simulink subsystem "PvtSubSys_HMI"  (R2020b)
settings: Solver=VariableStepAuto  StartTime=0.0  StopTime=10.0  RelTol=1e-3
undefined symbols (not defined in the file): P_HMI_LDW_LKAWarnTime, P_HMI_ObjectTypeFilter, P_HMI_WarnFormLDWReq
libraries: simulink x212, TrueDurationTime x6
(part 7 of 8)

== matlab function PvtSubSys_HMI/HMI2.12/HWA//ACC//TJA_Signal1/MATLAB Function7 ==
  data: AngRaw input single; Angle output single
function Angle = AngCalc(AngRaw)
if AngRaw>1.57
    Angle = AngRaw - single(3.14);
elseif AngRaw<-1.57
    Angle = AngRaw + single(3.14);
else
    Angle = AngRaw;
end

== matlab function PvtSubSys_HMI/HMI2.12/HWA//ACC//TJA_Signal1/MATLAB Function8 ==
  data: Lane_ChangeReq input; LaneChange output
function LaneChange = fcn(Lane_ChangeReq)
LaneChange=uint8(0);
if Lane_ChangeReq==1
    LaneChange=uint8(1);
elseif Lane_ChangeReq==2
    LaneChange=uint8(2);
end

== matlab function PvtSubSys_HMI/HMI2.12/IFC_Signal1/MATLAB Function ==
  data: ELKState input; ELKmainState output
function ELKmainState  = fcn(ELKState)
ELKmainState=ELKState;
if ELKState == 3 || ELKState == 4
    ELKmainState = uint8(3);
elseif ELKState == 5 ||  ELKState == 6
    ELKmainState =uint8(4);
elseif ELKState == 7 ||  ELKState == 8
    ELKmainState = uint8(5);
elseif ELKState == 9
    ELKmainState = uint8(6);
end

== matlab function PvtSubSys_HMI/HMI2.12/IFC_Signal1/MATLAB Function1 ==
  data: fType input; Type output
function Type = fcn(fType)

Type=fType;
if fType==14||fType==20
    Type=uint8(2);
end

== matlab function PvtSubSys_HMI/HMI2.12/IFC_Signal1/MATLAB Function10 ==
  data: Lvalid input; y output; Rvalid input
function y = fcn(Lvalid,Rvalid)
if Lvalid>1 && Rvalid>1
  y=3;%double
elseif Lvalid>1 && Rvalid<2
    y=1 ; % left
elseif Lvalid<2 && Rvalid>1
    y=2; %right
else 
    y=0;
end

== matlab function PvtSubSys_HMI/HMI2.12/IFC_Signal1/MATLAB Function11 ==
  data: ELKSts input; LDW_LKAWarn output; LKAState input; Time input; count output; countk1 input
function [LDW_LKAWarn,count] = fcn(ELKSts,LKAState,Time,countk1)
count=0;
LDW_LKAWarn=uint8(0);
if ELKSts==uint8(3)||ELKSts==uint8(5)||ELKSts==uint8(7) || LKAState==uint8(4)
    count=countk1+1;
    if countk1>50*(Time-1)
        
        LDW_LKAWarn=uint8(1);
    end
elseif ELKSts==uint8(4)||ELKSts==uint8(6)||ELKSts==uint8(8) || LKAState==uint8(5)
    count=countk1+1;
    if countk1>50*(Time-1)
        LDW_LKAWarn=uint8(2);
    end
end

== matlab function PvtSubSys_HMI/HMI2.12/IFC_Signal1/Subsystem1/MATLAB Function3 ==
  data: Left_A0 input; Left_A1 input; Left_A2 input; Left_A3 input; L_A0 output; L_A1 output; L_A2 output; L_A3 output; Left_Type input; Left_Valid input; Right_A0 input; Right_A1 input; Right_A2 input; Right_A3 input; Right_Type input; Right_Valid input; LaneAvailability input; L_Type output uint8; L_Valid output uint8; R_A0 output; R_A1 output; R_A2 output; R_A3 output; R_Type output uint8; R_Valid output uint8
function [L_A0,L_A1,L_A2,L_A3,L_Type,L_Valid,R_A0,R_A1,R_A2,R_A3,R_Type,R_Valid] = LineCalc(Left_A0,Left_A1,Left_A2,Left_A3......
,Left_Type,Left_Valid,Right_A0,Right_A1,Right_A2,Right_A3,Right_Type,Right_Valid,LaneAvailability)
L_A0=single(0);
L_A1=single(0);
L_A2=single(0);
L_A3=single(0);
L_Type=uint8(0);
L_Valid=uint8(1);
R_A0=single(0);
R_A1=single(0);
R_A2=single(0);
R_A3=single(0);
R_Type=uint8(0);
R_Valid=uint8(1);

if LaneAvailability==1
    L_A0=Left_A0;
    L_A1=Left_A1;
    L_A2=Left_A2;
    L_A3=Left_A3;
    L_Type=Left_Type;
    L_Valid=Left_Valid;
elseif LaneAvailability==2
    R_A0=Right_A0;
    R_A1=Right_A1;
    R_A2=Right_A2;
    R_A3=Right_A3;
    R_Type=Right_Type;
    R_Valid=Right_Valid;
elseif LaneAvailability==3
    if abs(Left_A0-Right_A0)<5.5 && abs(Left_A0-Right_A0)>2.5
        L_A0=Left_A0;
        L_A1=Left_A1;
        L_A2=Left_A2;
        L_A3=Left_A3;
        L_Type=Left_Type;
        L_Valid=Left_Valid;
        R_A0=Right_A0;
        R_A1=Right_A1;
        R_A2=Right_A2;
        R_A3=Right_A3;
        R_Type=Right_Type;
        R_Valid=Right_Valid;
    elseif abs(Left_A0-Right_A0)>=5.5
        L_A0=5.5*Left_A0/abs(Left_A0-Right_A0);
        L_A1=Left_A1;
        L_A2=Left_A2;
        L_A3=Left_A3;
        L_Type=Left_Type;
        L_Valid=Left_Valid;
        R_A0=5.5*Right_A0/abs(Left_A0-Right_A0);
        R_A1=Right_A1;
        R_A2=Right_A2;
        R_A3=Right_A3;
        R_Type=Right_Type;
        R_Valid=Right_Valid;
    elseif abs(Left_A0-Right_A0)<=2.5&&abs(Left_A0-Right_A0)>0
        L_A0=2.5*Left_A0/abs(Left_A0-Right_A0);
        L_A1=Left_A1;
        L_A2=Left_A2;
        L_A3=Left_A3;
        L_Type=Left_Type;
        L_Valid=Left_Valid;
        R_A0=2.5*Right_A0/abs(Left_A0-Right_A0);
        R_A1=Right_A1;
        R_A2=Right_A2;
        R_A3=Right_A3;
        R_Type=Right_Type;
        R_Valid=Right_Valid;
    end
end

== matlab function PvtSubSys_HMI/HMI2.12/IFC_Signal1/MATLAB Function4 ==
  data: fType input; Type output
function Type = fcn(fType)

Type=fType;
if fType==14||fType==20
    Type=uint8(2);
end

== matlab function PvtSubSys_HMI/HMI2.12/IFC_Signal1/MATLAB Function5 ==
  data: fType input; Type output
function Type = fcn(fType)

Type=fType;
if fType==14||fType==20
    Type=uint8(2);
end

== matlab function PvtSubSys_HMI/HMI2.12/IFC_Signal1/Subsystem53/MATLAB Function1 ==
  data: standstill input boolean; out output single; in input single; update input boolean; inrecorder input single; recorder output single
function [out,recorder] = fcn(standstill,in,update,inrecorder)
recorder=inrecorder;
out=single(0);
if update%当车辆由运动到静止时记录recorder，并在车辆运动时将recorder清零
    recorder=in;
end
if standstill==0%车辆运动时采用实际值，车辆静止时采用recorder值
    out=in;
elseif standstill==1
    if update
        out=in;
    else
        out=inrecorder;
    end
end

== matlab function PvtSubSys_HMI/HMI2.12/IFC_Signal1/MATLAB Function7 ==
  data: ESSSts input; Intervention output; State output; Error output
function [Intervention,State,Error]  = fcn(ESSSts)

Intervention=uint8(0);
State=uint8(0);
Error=false;
if ESSSts>0
    State=uint8(1);
end
if ESSSts==4
    Intervention=uint8(1);
elseif ESSSts==5
    Intervention=uint8(2);
elseif ESSSts==6
    Error=true;
end

== matlab function PvtSubSys_HMI/HMI2.12/IFC_Signal1/MATLAB Function8 ==
  data: LDWActive input; LSSIntervention input; warnform input; WarnFormReq input; y output
function y = fcn(LDWActive, LSSIntervention,warnform, WarnFormReq)
y=uint8(0);
if (LSSIntervention==1 || LSSIntervention==2 || LSSIntervention==6 || LSSIntervention==7) && warnform==0
    if WarnFormReq==1 || WarnFormReq==2
        y=uint8(1);
    end
elseif (LSSIntervention==1 || LSSIntervention==2 || LSSIntervention==6 || LSSIntervention==7) && warnform==1
    if (WarnFormReq==1 || WarnFormReq==2) && LDWActive==true
        y=uint8(1);
    end   
end

== matlab function PvtSubSys_HMI/HMI2.12/IFC_Signal1/MATLAB Function9 ==
  data: ESSSts input; Intervention output; State output; Error output
function [Intervention,State,Error]  = fcn(ESSSts)

Intervention=uint8(0);
State=uint8(0);
Error=false;
if ESSSts>0
    State=uint8(1);
end
if ESSSts==4
    Intervention=uint8(1);
elseif ESSSts==5
    Intervention=uint8(2);
elseif ESSSts==6
    Error=true;
end

== matlab function PvtSubSys_HMI/HMI2.12/HWA//ACC//TJA_Signal1/MATLAB Function9 ==
  data: IntelligentCurveActive input boolean; y output uint8; ISL_InterSysInfoDisp input uint8; yk1 input uint8; countk1 input single; count output single
function [y,count] = fcn(IntelligentCurveActive, ISL_InterSysInfoDisp,yk1,countk1)

if yk1==uint8(3)
    count=single(6000);
else
    count=max(single(0),countk1-single(1));
end
if IntelligentCurveActive==true && count==single(0)
    y=uint8(3);
elseif ISL_InterSysInfoDisp==1 || ISL_InterSysInfoDisp==2 
    y=ISL_InterSysInfoDisp;
else
    y=uint8(0);
end

== matlab function PvtSubSys_HMI/HMI2.12/IFC_Signal1/Subsystem1/MATLAB Function2 ==
  data: LeftValid input; LaneAvailability output; RightValid input; LeftA0 input; RightA0 input
function LaneAvailability = fcn(LeftValid,RightValid,LeftA0,RightA0)
LaneAvailability=0;
if LeftValid==true && RightValid== true %% two lane
    LaneAvailability=3;
elseif LeftValid==true && RightValid==false %% left lane
    LaneAvailability=1;
elseif LeftValid==false && RightValid==true %% right lane
    LaneAvailability=2;
end

== matlab function PvtSubSys_HMI/HMI2.12/IFC_Signal1/Subsystem2/MATLAB Function ==
  data: Left_A0 input; L_A0 output; Left_Type input; Right_A0 input; Right_Type input; LaneAvailability input; L_Type output; R_A0 output; R_Type output
function [L_A0,L_Type,R_A0,R_Type] = fcn(Left_A0,Left_Type,Right_A0,Right_Type,LaneAvailability)
    L_A0=single(0);
    R_A0=single(0);
    L_Type=uint8(0);
    R_Type=uint8(0);
    
if LaneAvailability==1
    L_A0=Left_A0; 
    L_Type=Left_Type;
elseif LaneAvailability==2
    R_A0=Right_A0;
    R_Type=Right_Type;
elseif LaneAvailability==3
    L_A0=Left_A0;
    L_Type=Left_Type;
    R_A0=Right_A0;
    R_Type=Right_Type;
end

== matlab function PvtSubSys_HMI/HMI2.12/IFC_Signal1/Subsystem2/MATLAB Function2 ==
  data: LeftValid input; LeftA0 input; LaneAvailability output; RightValid input; RightA0 input
function LaneAvailability = fcn(LeftValid,LeftA0,RightValid,RightA0)

 LaneAvailability=0;
if LeftValid==true && RightValid== true %% two lane
    if LeftA0-RightA0>=5.5
        LaneAvailability=0;
        if LeftA0 < 2.75
            LaneAvailability=1;
        elseif RightA0> -2.75
            LaneAvailability=2;
        end
    elseif LeftA0-RightA0<5.5 && LeftA0-RightA0>2.5
         LaneAvailability=3;
    end
elseif LeftValid==true && RightValid==false %% left lane
    if LeftA0<2.75
        LaneAvailability=1;
    end
elseif LeftValid==false && RightValid==true %% right lane
    if RightA0>-2.75
         LaneAvailability=2;
    end
end

== matlab function PvtSubSys_HMI/HMI2.12/IFC_Signal1/MATLAB Function2 ==
  data: LSSSwtReq input; LDWState input; LKAState input; LCKState input; ELKSts input; LKAWarning input; LCKIESts input; TJAState input; LSS_WarnFormSwtReq input; LKASwtReq input; LCKSwtReq input; Lcountk1 input; LSSFuncSts output; LSSErrSts output; LSSResp output; LSSIntervention output; ELKResp output; LCKResp output; LKAResp output; LDWResp output; IntelligentEvaResp output; IntelligentEvaActSts output; Lcount output; Rcountk1 input; Rcount output
function [LSSFuncSts,LSSErrSts,LSSResp,LSSIntervention,ELKResp,LCKResp,LKAResp,LDWResp,......
    IntelligentEvaResp,IntelligentEvaActSts,Lcount,Rcount] = fcn( LSSSwtReq,LDWState,LKAState,LCKState,ELKSts,LKAWarning,LCKIESts,TJAState,LSS_WarnFormSwtReq,LKASwtReq,LCKSwtReq,Lcountk1,Rcountk1)
LSSIntervention=uint8(0);
LSSErrSts=uint8(0);
LSSResp=false;
LSSFuncSts=uint8(0);
ELKResp=false;
LCKResp=false;
LKAResp=false;
LDWResp=false;
IntelligentEvaResp=false;
IntelligentEvaActSts=uint8(0);
Lcount=50;
Rcount=50;


%% LSSSwtReq
if LSSSwtReq>0
     LSSResp=true;
end


%% LCKState
    if LCKState>0 && LCKSwtReq>0
        LCKResp=true;
        LSSFuncSts=uint8(3);
        if LCKState==3 && (ELKSts==0||ELKSts==1||ELKSts==2||ELKSts==9 || LKAState~=4 || LKAState~=5)
            LSSIntervention=uint8(5);
            if LKAWarning==1
                if LSS_WarnFormSwtReq==0 || LSS_WarnFormSwtReq==2
                LSSIntervention=uint8(1);
                elseif LSS_WarnFormSwtReq==1
                LSSIntervention=uint8(6);
                end
            elseif LKAWarning==2
               if LSS_WarnFormSwtReq==0 ||  LSS_WarnFormSwtReq==2
                  LSSIntervention=uint8(2);
               elseif LSS_WarnFormSwtReq==1
                LSSIntervention=uint8(7);
               end
            end
                
        elseif LCKState==7
            LSSErrSts=uint8(3);
        end
        
 %% LKAState
    elseif LKAState>0 &&  LKASwtReq>0
        LKAResp=true;
        LSSFuncSts=uint8(2);
        if LKAState==4 && (ELKSts==0||ELKSts==1||ELKSts==2||ELKSts==9)|| (Lcountk1>0&&Lcountk1<50)
            Lcount=max(0,Lcountk1-1);
            LSSIntervention=uint8(3);
            if LKAWarning==1 
                if LSS_WarnFormSwtReq==0 || LSS_WarnFormSwtReq==2
                LSSIntervention=uint8(1);
                elseif LSS_WarnFormSwtReq==1
                LSSIntervention=uint8(6);
                end
            end
        elseif LKAState==5 && (ELKSts==0||ELKSts==1||ELKSts==2||ELKSts==9)|| (Rcountk1>0&&Rcountk1<50)
            Rcount=max(0,Lcountk1-1);
            LSSIntervention=uint8(4);
            if LKAWarning==1
               if LSS_WarnFormSwtReq==0 ||  LSS_WarnFormSwtReq==2
                  LSSIntervention=uint8(2);
               elseif LSS_WarnFormSwtReq==1
                LSSIntervention=uint8(7);
               end
            end
        elseif LKAState==6
            LSSErrSts=uint8(2);
        end
%%  LDWState
    elseif LDWState>0
        LSSFuncSts=uint8(1);
        LDWResp=true;
        if LDWState==4 && (ELKSts==0||ELKSts==1||ELKSts==2||ELKSts==9|| LKAState~=4 || LKAState~=5)
            if LSS_WarnFormSwtReq==0 || LSS_WarnFormSwtReq==2
            LSSIntervention=uint8(1);
            elseif LSS_WarnFormSwtReq==1
                LSSIntervention=uint8(6);
            end
        elseif LDWState==5 && (ELKSts==0||ELKSts==1||ELKSts==2||ELKSts==9|| LKAState~=4 || LKAState~=5)
            if LSS_WarnFormSwtReq==0 ||  LSS_WarnFormSwtReq==2
            LSSIntervention=uint8(2);
            elseif LSS_WarnFormSwtReq==1
                LSSIntervention=uint8(7);
            end
        elseif LDWState==6 
            LSSErrSts=uint8(1);
        end   
    end
   

%% LCKIESwitch
if LCKIESts>0
    IntelligentEvaResp=true;
    if LCKIESts==4
        IntelligentEvaActSts=uint8(2);
    elseif LCKIESts==5
        IntelligentEvaActSts=uint8(1);
    end
end
%% ELKState
if ELKSts>0
   ELKResp=true;
   LSSFuncSts=uint8(2);
   if LCKState>0 && LCKSwtReq>0
       LSSFuncSts=uint8(3);
   end
    if ELKSts==5 || ELKSts==7 || ELKSts==3
            LSSIntervention=uint8(3);
            if LKAWarning==1
                if LSS_WarnFormSwtReq==0 || LSS_WarnFormSwtReq==2
                LSSIntervention=uint8(1);
                elseif LSS_WarnFormSwtReq==1
                LSSIntervention=uint8(6);
                end
            end
    elseif ELKSts==6 || ELKSts==8 || ELKSts==4
            LSSIntervention=uint8(4);
            if LKAWarning==1
               if LSS_WarnFormSwtReq==0 ||  LSS_WarnFormSwtReq==2
                  LSSIntervention=uint8(2);
               elseif LSS_WarnFormSwtReq==1
                LSSIntervention=uint8(7);
               end
            end
    elseif LKAState==4 || (Lcountk1>0&&Lcountk1<50)
         Lcount=max(0,Lcountk1-1);
            LSSIntervention=uint8(3);
            if LKAWarning==1 
                if LSS_WarnFormSwtReq==0 || LSS_WarnFormSwtReq==2
                LSSIntervention=uint8(1);
                elseif LSS_WarnFormSwtReq==1
                LSSIntervention=uint8(6);
                end
            end
    elseif LKAState==5 || (Rcountk1>0&&Rcountk1<50)
        Rcount=max(0,Lcountk1-1);
            LSSIntervention=uint8(4);
            if LKAWarning==1
               if LSS_WarnFormSwtReq==0 ||  LSS_WarnFormSwtReq==2
                  LSSIntervention=uint8(2);
               elseif LSS_WarnFormSwtReq==1
                LSSIntervention=uint8(7);
               end
            end
    elseif LCKState~=7 && LKAState~=6 && ELKSts==9
        LSSErrSts=uint8(4);
    end
end
%% TJAState
if ((TJAState==3 || TJAState==9 || TJAState==10)&& LCKState==3)
     LSSIntervention=uint8(5);

end

== matlab function PvtSubSys_HMI/HMI2.12/IFC_Signal1/MATLAB Function12 ==
  data: ELKState input; ELKActSts output
function ELKActSts  = fcn(ELKState)
ELKActSts=uint8(0);
if ELKState==uint8(3) || ELKState==uint8(5) || ELKState==uint8(7)
    ELKActSts=uint8(1);
elseif ELKState==uint8(4) || ELKState==uint8(6) || ELKState==uint8(8)
    ELKActSts=uint8(2);
end

== matlab function PvtSubSys_HMI/HMI2.12/IFC_Signal1/MATLAB Function3 ==
  data: LSSSwtReq input; LDWState input; LKAState input; LCKState input; ELKSts input; LKAWarning input; LCKIESts input; TJAState input; LSS_WarnFormSwtReq input; LKASwtReq input; LCKSwtReq input; Lcountk1 input; LSSFuncSts output; LSSErrSts output; LSSResp output; LSSIntervention output; ELKResp output; LCKResp output; LKAResp output; LDWResp output; IntelligentEvaResp output; IntelligentEvaActSts output; Lcount output; Rcountk1 input; Rcount output
function [LSSFuncSts,LSSErrSts,LSSResp,LSSIntervention,ELKResp,LCKResp,LKAResp,LDWResp,......
    IntelligentEvaResp,IntelligentEvaActSts,Lcount,Rcount] = fcn( LSSSwtReq,LDWState,LKAState,LCKState,ELKSts,LKAWarning,LCKIESts,TJAState,LSS_WarnFormSwtReq,LKASwtReq,LCKSwtReq,Lcountk1,Rcountk1)
LSSIntervention=uint8(0);
LSSErrSts=uint8(0);
LSSResp=false;
LSSFuncSts=uint8(0);
ELKResp=false;
LCKResp=false;
LKAResp=false;
LDWResp=false;
IntelligentEvaResp=false;
IntelligentEvaActSts=uint8(0);
Lcount=50;
Rcount=50;


%% LSSSwtReq
if LSSSwtReq>0
     LSSResp=true;
end


%% LCKState
    if LCKState>0 && LCKSwtReq>0
        LCKResp=true;
        LSSFuncSts=uint8(3);
        if LCKState==3 && (ELKSts==0||ELKSts==1||ELKSts==2||ELKSts==9 || LKAState~=4 || LKAState~=5)
            LSSIntervention=uint8(5);
            if LKAWarning==1
                if LSS_WarnFormSwtReq==0 || LSS_WarnFormSwtReq==2
                LSSIntervention=uint8(1);
                elseif LSS_WarnFormSwtReq==1
                LSSIntervention=uint8(6);
                end
            elseif LKAWarning==2
               if LSS_WarnFormSwtReq==0 ||  LSS_WarnFormSwtReq==2
                  LSSIntervention=uint8(2);
               elseif LSS_WarnFormSwtReq==1
                LSSIntervention=uint8(7);
               end
            end
                
        elseif LCKState==7
            LSSErrSts=uint8(3);
        end
        
 %% LKAState
    elseif LKAState>0 &&  LKASwtReq>0
        LKAResp=true;
        LSSFuncSts=uint8(2);
        if (LKAState==4|| (Lcountk1>0&&Lcountk1<50)) && (ELKSts==0||ELKSts==1||ELKSts==2||ELKSts==9)
            Lcount=max(0,Lcountk1-1);
            LSSIntervention=uint8(3);
            if LKAWarning==1 
                if LSS_WarnFormSwtReq==0 || LSS_WarnFormSwtReq==2
                LSSIntervention=uint8(1);
                elseif LSS_WarnFormSwtReq==1
                LSSIntervention=uint8(6);
                end
            end
        elseif (LKAState==5|| (Rcountk1>0&&Rcountk1<50)) && (ELKSts==0||ELKSts==1||ELKSts==2||ELKSts==9)
            Rcount=max(0,Lcountk1-1);
            LSSIntervention=uint8(4);
            if LKAWarning==1
               if LSS_WarnFormSwtReq==0 ||  LSS_WarnFormSwtReq==2
                  LSSIntervention=uint8(2);
               elseif LSS_WarnFormSwtReq==1
                LSSIntervention=uint8(7);
               end
            end
        elseif LKAState==6
            LSSErrSts=uint8(2);
        end
%%  LDWState
    elseif LDWState>0
        LSSFuncSts=uint8(1);
        LDWResp=true;
        if LDWState==4 && (ELKSts==0||ELKSts==1||ELKSts==2||ELKSts==9|| LKAState~=4 || LKAState~=5)
            if LSS_WarnFormSwtReq==0 || LSS_WarnFormSwtReq==2
            LSSIntervention=uint8(1);
            elseif LSS_WarnFormSwtReq==1
                LSSIntervention=uint8(6);
            end
        elseif LDWState==5 && (ELKSts==0||ELKSts==1||ELKSts==2||ELKSts==9|| LKAState~=4 || LKAState~=5)
            if LSS_WarnFormSwtReq==0 ||  LSS_WarnFormSwtReq==2
            LSSIntervention=uint8(2);
            elseif LSS_WarnFormSwtReq==1
                LSSIntervention=uint8(7);
            end
        elseif LDWState==6 
            LSSErrSts=uint8(1);
        end   
    end
   

%% LCKIESwitch
if LCKIESts>0
    IntelligentEvaResp=true;
    if LCKIESts==4
        IntelligentEvaActSts=uint8(2);
    elseif LCKIESts==5
        IntelligentEvaActSts=uint8(1);
    end
end
%% ELKState
if ELKSts>0
   ELKResp=true;
   LSSFuncSts=uint8(2);
   if LCKState>0 && LCKSwtReq>0
       LSSFuncSts=uint8(3);
   end
    if ELKSts==5 || ELKSts==7 || ELKSts==3
            LSSIntervention=uint8(3);
            if LKAWarning==1
                if LSS_WarnFormSwtReq==0 || LSS_WarnFormSwtReq==2
                LSSIntervention=uint8(1);
                elseif LSS_WarnFormSwtReq==1
                LSSIntervention=uint8(6);
                end
            end
    elseif ELKSts==6 || ELKSts==8 || ELKSts==4
            LSSIntervention=uint8(4);
            if LKAWarning==1
               if LSS_WarnFormSwtReq==0 ||  LSS_WarnFormSwtReq==2
                  LSSIntervention=uint8(2);
               elseif LSS_WarnFormSwtReq==1
                LSSIntervention=uint8(7);
               end
            end
    elseif LKAState==4 || (Lcountk1>0&&Lcountk1<50)
         Lcount=max(0,Lcountk1-1);
            LSSIntervention=uint8(3);
            if LKAWarning==1 
                if LSS_WarnFormSwtReq==0 || LSS_WarnFormSwtReq==2
                LSSIntervention=uint8(1);
                elseif LSS_WarnFormSwtReq==1
                LSSIntervention=uint8(6);
                end
            end
    elseif LKAState==5 || (Rcountk1>0&&Rcountk1<50)
        Rcount=max(0,Lcountk1-1);
            LSSIntervention=uint8(4);
            if LKAWarning==1
               if LSS_WarnFormSwtReq==0 ||  LSS_WarnFormSwtReq==2
                  LSSIntervention=uint8(2);
               elseif LSS_WarnFormSwtReq==1
                LSSIntervention=uint8(7);
               end
            end
    elseif LCKState~=7 && LKAState~=6 && ELKSts==9
        LSSErrSts=uint8(4);
    end
end
%% TJAState
if ((TJAState==3 || TJAState==9 || TJAState==10)&& LCKState==3)
     LSSIntervention=uint8(5);

end

== matlab function PvtSubSys_HMI/MATLAB Function1 ==
  data: Le1LineExist input; A1 output; Ri1LineExist input; Le1C1 input; Le1C2 input; Le1C3 input; Ri1C1 input; Ri1C2 input; Ri1C3 input; A2 output; A3 output; LB_Exist input; LB_C1 input; LB_C2 input; LB_C3 input; RB_Exist input; RB_C1 input; RB_C2 input; RB_C3 input
function [A1,A2,A3] = ...
    LineTranCalc(Le1LineExist,Ri1LineExist,...
    Le1C1,Le1C2,Le1C3,Ri1C1,Ri1C2,Ri1C3,LB_Exist,LB_C1,LB_C2,LB_C3,RB_Exist,RB_C1,RB_C2,RB_C3)

if Le1LineExist==uint8(2) && Ri1LineExist==uint8(2)
    A1 = 0.5*Le1C1 + 0.5*Ri1C1;
    A2 = 0.5*Le1C2 + 0.5*Ri1C2;
    A3 = 0.5*Le1C3 + 0.5*Ri1C3;
elseif Le1LineExist==uint8(2)
    A1 = Le1C1;
    A2 = Le1C2;
    A3 = Le1C3;
elseif Ri1LineExist==uint8(2)
    A1 = Ri1C1;
    A2 = Ri1C2;
    A3 = Ri1C3;
elseif LB_Exist==uint8(2) && RB_Exist==uint8(2)
    A1 = 0.5*LB_C1 + 0.5*RB_C1;
    A2 = 0.5*LB_C2 + 0.5*RB_C2;
    A3 = 0.5*LB_C3 + 0.5*RB_C3;
elseif LB_Exist==uint8(2)
    A1 = LB_C1;
    A2 = LB_C2;
    A3 = LB_C3;
elseif RB_Exist==uint8(2)
    A1 = RB_C1;
    A2 = RB_C2;
    A3 = RB_C3;
else
    A1 = single(0);
    A2 = single(0);
    A3 = single(0);
end

== matlab function PvtSubSys_HMI/HMI2.12/IFC_Signal1/Subsystem4/MATLAB Function1 ==
  data: standstill input boolean; out output uint8; in input uint8; update input boolean; inrecorder input uint8; recorder output uint8
function [out,recorder] = fcn(standstill,in,update,inrecorder)
recorder=inrecorder;
out=uint8(0);
if update%当车辆由运动到静止时记录recorder，并在车辆运动时将recorder清零
    recorder=in;
end
if standstill==0%车辆运动时采用实际值，车辆静止时采用recorder值
    out=in;
elseif standstill==1
    if update
        out=in;
    else
        out=inrecorder;
    end
end

== matlab function PvtSubSys_HMI/HMI2.12/IFC_Signal1/Subsystem3/MATLAB Function1 ==
  data: standstill input boolean; out output uint8; in input uint8; update input boolean; inrecorder input uint8; recorder output uint8
function [out,recorder] = fcn(standstill,in,update,inrecorder)
recorder=inrecorder;
out=uint8(0);
if update%当车辆由运动到静止时记录recorder，并在车辆运动时将recorder清零
    recorder=in;
end
if standstill==0%车辆运动时采用实际值，车辆静止时采用recorder值
    out=in;
elseif standstill==1
    if update
        out=in;
    else
        out=inrecorder;
    end
end

== matlab function PvtSubSys_HMI/HMI2.12/IFC_Signal1/Subsystem5/MATLAB Function1 ==
  data: standstill input boolean; out output uint8; in input uint8; update input boolean; inrecorder input uint8; recorder output uint8
function [out,recorder] = fcn(standstill,in,update,inrecorder)
recorder=inrecorder;
out=uint8(0);
if update%当车辆由运动到静止时记录recorder，并在车辆运动时将recorder清零
    recorder=in;
end
if standstill==0%车辆运动时采用实际值，车辆静止时采用recorder值
    out=in;
elseif standstill==1
    if update
        out=in;
    else
        out=inrecorder;
    end
end

== matlab function PvtSubSys_HMI/HMI2.12/IFC_Signal1/Subsystem6/MATLAB Function1 ==
  data: standstill input boolean; out output uint8; in input uint8; update input boolean; inrecorder input uint8; recorder output uint8
function [out,recorder] = fcn(standstill,in,update,inrecorder)
recorder=inrecorder;
out=uint8(0);
if update%当车辆由运动到静止时记录recorder，并在车辆运动时将recorder清零
    recorder=in;
end
if standstill==0%车辆运动时采用实际值，车辆静止时采用recorder值
    out=in;
elseif standstill==1
    if update
        out=in;
    else
        out=inrecorder;
    end
end

== matlab function PvtSubSys_HMI/HMI2.12/IFC_Signal1/Subsystem7/MATLAB Function1 ==
  data: standstill input boolean; out output uint8; in input uint8; update input boolean; inrecorder input uint8; recorder output uint8
function [out,recorder] = fcn(standstill,in,update,inrecorder)
recorder=inrecorder;
out=uint8(0);
if update%当车辆由运动到静止时记录recorder，并在车辆运动时将recorder清零
    recorder=in;
end
if standstill==0%车辆运动时采用实际值，车辆静止时采用recorder值
    out=in;
elseif standstill==1
    if update
        out=in;
    else
        out=inrecorder;
    end
end

== matlab function PvtSubSys_HMI/HMI2.12/IFC_Signal1/Subsystem8/MATLAB Function1 ==
  data: standstill input boolean; out output uint8; in input uint8; update input boolean; inrecorder input uint8; recorder output uint8
function [out,recorder] = fcn(standstill,in,update,inrecorder)
recorder=inrecorder;
out=uint8(0);
if update%当车辆由运动到静止时记录recorder，并在车辆运动时将recorder清零
    recorder=in;
end
if standstill==0%车辆运动时采用实际值，车辆静止时采用recorder值
    out=in;
elseif standstill==1
    if update
        out=in;
    else
        out=inrecorder;
    end
end

== matlab function PvtSubSys_HMI/HMI2.12/IFC_Signal1/Subsystem9/MATLAB Function1 ==
  data: standstill input boolean; out output uint8; in input uint8; update input boolean; inrecorder input uint8; recorder output uint8
function [out,recorder] = fcn(standstill,in,update,inrecorder)
recorder=inrecorder;
out=uint8(0);
if update%当车辆由运动到静止时记录recorder，并在车辆运动时将recorder清零
    recorder=in;
end
if standstill==0%车辆运动时采用实际值，车辆静止时采用recorder值
    out=in;
elseif standstill==1
    if update
        out=in;
    else
        out=inrecorder;
    end
end

== matlab function PvtSubSys_HMI/HMI2.12/IFC_Signal1/Subsystem10/MATLAB Function1 ==
  data: standstill input boolean; out output uint8; in input uint8; update input boolean; inrecorder input uint8; recorder output uint8
function [out,recorder] = fcn(standstill,in,update,inrecorder)
recorder=inrecorder;
out=uint8(0);
if update%当车辆由运动到静止时记录recorder，并在车辆运动时将recorder清零
    recorder=in;
end
if standstill==0%车辆运动时采用实际值，车辆静止时采用recorder值
    out=in;
elseif standstill==1
    if update
        out=in;
    else
        out=inrecorder;
    end
end

== matlab function PvtSubSys_HMI/HMI2.12/IFC_Signal1/Subsystem11/MATLAB Function1 ==
  data: standstill input boolean; out output single; in input single; update input boolean; inrecorder input single; recorder output single
function [out,recorder] = fcn(standstill,in,update,inrecorder)
recorder=inrecorder;
out=single(0);
if update%当车辆由运动到静止时记录recorder，并在车辆运动时将recorder清零
    recorder=in;
end
if standstill==0%车辆运动时采用实际值，车辆静止时采用recorder值
    out=in;
elseif standstill==1
    if update
        out=in;
    else
        out=inrecorder;
    end
end

== matlab function PvtSubSys_HMI/HMI2.12/IFC_Signal1/Subsystem12/MATLAB Function1 ==
  data: standstill input boolean; out output single; in input single; update input boolean; inrecorder input single; recorder output single
function [out,recorder] = fcn(standstill,in,update,inrecorder)
recorder=inrecorder;
out=single(0);
if update%当车辆由运动到静止时记录recorder，并在车辆运动时将recorder清零
    recorder=in;
end
if standstill==0%车辆运动时采用实际值，车辆静止时采用recorder值
    out=in;
elseif standstill==1
    if update
        out=in;
    else
        out=inrecorder;
    end
end

== matlab function PvtSubSys_HMI/HMI2.12/IFC_Signal1/Subsystem13/MATLAB Function1 ==
  data: standstill input boolean; out output uint8; in input uint8; update input boolean; inrecorder input uint8; recorder output uint8
function [out,recorder] = fcn(standstill,in,update,inrecorder)
recorder=inrecorder;
out=uint8(0);
if update%当车辆由运动到静止时记录recorder，并在车辆运动时将recorder清零
    recorder=in;
end
if standstill==0%车辆运动时采用实际值，车辆静止时采用recorder值
    out=in;
elseif standstill==1
    if update
        out=in;
    else
        out=inrecorder;
    end
end

== matlab function PvtSubSys_HMI/HMI2.12/IFC_Signal1/Subsystem14/MATLAB Function1 ==
  data: standstill input boolean; out output uint8; in input uint8; update input boolean; inrecorder input uint8; recorder output uint8
function [out,recorder] = fcn(standstill,in,update,inrecorder)
recorder=inrecorder;
out=uint8(0);
if update%当车辆由运动到静止时记录recorder，并在车辆运动时将recorder清零
    recorder=in;
end
if standstill==0%车辆运动时采用实际值，车辆静止时采用recorder值
    out=in;
elseif standstill==1
    if update
        out=in;
    else
        out=inrecorder;
    end
end

== matlab function PvtSubSys_HMI/HMI2.12/IFC_Signal1/Subsystem15/MATLAB Function1 ==
  data: standstill input boolean; out output single; in input single; update input boolean; inrecorder input single; recorder output single
function [out,recorder] = fcn(standstill,in,update,inrecorder)
recorder=inrecorder;
out=single(0);
if update%当车辆由运动到静止时记录recorder，并在车辆运动时将recorder清零
    recorder=in;
end
if standstill==0%车辆运动时采用实际值，车辆静止时采用recorder值
    out=in;
elseif standstill==1
    if update
        out=in;
    else
        out=inrecorder;
    end
end

== matlab function PvtSubSys_HMI/HMI2.12/IFC_Signal1/Subsystem16/MATLAB Function1 ==
  data: standstill input boolean; out output single; in input single; update input boolean; inrecorder input single; recorder output single
function [out,recorder] = fcn(standstill,in,update,inrecorder)
recorder=inrecorder;
out=single(0);
if update%当车辆由运动到静止时记录recorder，并在车辆运动时将recorder清零
    recorder=in;
end
if standstill==0%车辆运动时采用实际值，车辆静止时采用recorder值
    out=in;
elseif standstill==1
    if update
        out=in;
    else
        out=inrecorder;
    end
end

== matlab function PvtSubSys_HMI/HMI2.12/IFC_Signal1/Subsystem17/MATLAB Function1 ==
  data: standstill input boolean; out output single; in input single; update input boolean; inrecorder input single; recorder output single
function [out,recorder] = fcn(standstill,in,update,inrecorder)
recorder=inrecorder;
out=single(0);
if update%当车辆由运动到静止时记录recorder，并在车辆运动时将recorder清零
    recorder=in;
end
if standstill==0%车辆运动时采用实际值，车辆静止时采用recorder值
    out=in;
elseif standstill==1
    if update
        out=in;
    else
        out=inrecorder;
    end
end

== matlab function PvtSubSys_HMI/HMI2.12/IFC_Signal1/Subsystem18/MATLAB Function1 ==
  data: standstill input boolean; out output single; in input single; update input boolean; inrecorder input single; recorder output single
function [out,recorder] = fcn(standstill,in,update,inrecorder)
recorder=inrecorder;
out=single(0);
if update%当车辆由运动到静止时记录recorder，并在车辆运动时将recorder清零
    recorder=in;
end
if standstill==0%车辆运动时采用实际值，车辆静止时采用recorder值
    out=in;
elseif standstill==1
    if update
        out=in;
    else
        out=inrecorder;
    end
end

== matlab function PvtSubSys_HMI/HMI2.12/IFC_Signal1/Subsystem19/MATLAB Function1 ==
  data: standstill input boolean; out output single; in input single; update input boolean; inrecorder input single; recorder output single
function [out,recorder] = fcn(standstill,in,update,inrecorder)
recorder=inrecorder;
out=single(0);
if update%当车辆由运动到静止时记录recorder，并在车辆运动时将recorder清零
    recorder=in;
end
if standstill==0%车辆运动时采用实际值，车辆静止时采用recorder值
    out=in;
elseif standstill==1
    if update
        out=in;
    else
        out=inrecorder;
    end
end

== matlab function PvtSubSys_HMI/HMI2.12/IFC_Signal1/Subsystem20/MATLAB Function1 ==
  data: standstill input boolean; out output single; in input single; update input boolean; inrecorder input single; recorder output single
function [out,recorder] = fcn(standstill,in,update,inrecorder)
recorder=inrecorder;
out=single(0);
if update%当车辆由运动到静止时记录recorder，并在车辆运动时将recorder清零
    recorder=in;
end
if standstill==0%车辆运动时采用实际值，车辆静止时采用recorder值
    out=in;
elseif standstill==1
    if update
        out=in;
    else
        out=inrecorder;
    end
end

== matlab function PvtSubSys_HMI/HMI2.12/IFC_Signal1/Subsystem21/MATLAB Function1 ==
  data: standstill input boolean; out output single; in input single; update input boolean; inrecorder input single; recorder output single
function [out,recorder] = fcn(standstill,in,update,inrecorder)
recorder=inrecorder;
out=single(0);
if update%当车辆由运动到静止时记录recorder，并在车辆运动时将recorder清零
    recorder=in;
end
if standstill==0%车辆运动时采用实际值，车辆静止时采用recorder值
    out=in;
elseif standstill==1
    if update
        out=in;
    else
        out=inrecorder;
    end
end

== matlab function PvtSubSys_HMI/HMI2.12/IFC_Signal1/Subsystem22/MATLAB Function1 ==
  data: standstill input boolean; out output single; in input single; update input boolean; inrecorder input single; recorder output single
function [out,recorder] = fcn(standstill,in,update,inrecorder)
recorder=inrecorder;
out=single(0);
if update%当车辆由运动到静止时记录recorder，并在车辆运动时将recorder清零
    recorder=in;
end
if standstill==0%车辆运动时采用实际值，车辆静止时采用recorder值
    out=in;
elseif standstill==1
    if update
        out=in;
    else
        out=inrecorder;
    end
end

== matlab function PvtSubSys_HMI/HMI2.12/HWA//ACC//TJA_Signal1/Enlong3s/MATLAB Function ==
  data: CntK1 input uint16; Cnt output uint16; X input; Num input
function Cnt= TextCount(CntK1,X,Num)

if X==true
    Cnt = Num;
else
     Cnt = max(CntK1-uint16(1),uint16(0));
end

== matlab function PvtSubSys_HMI/HMI2.12/IFC_Signal1/Subsystem23/MATLAB Function1 ==
  data: standstill input boolean; out output single; in input single; update input boolean; inrecorder input single; recorder output single
function [out,recorder] = fcn(standstill,in,update,inrecorder)
recorder=inrecorder;
out=single(0);
if update%当车辆由运动到静止时记录recorder，并在车辆运动时将recorder清零
    recorder=in;
end
if standstill==0%车辆运动时采用实际值，车辆静止时采用recorder值
    out=in;
elseif standstill==1
    if update
        out=in;
    else
        out=inrecorder;
    end
end

== matlab function PvtSubSys_HMI/HMI2.12/IFC_Signal1/Subsystem24/MATLAB Function1 ==
  data: standstill input boolean; out output single; in input single; update input boolean; inrecorder input single; recorder output single
function [out,recorder] = fcn(standstill,in,update,inrecorder)
recorder=inrecorder;
out=single(0);
if update%当车辆由运动到静止时记录recorder，并在车辆运动时将recorder清零
    recorder=in;
end
if standstill==0%车辆运动时采用实际值，车辆静止时采用recorder值
    out=in;
elseif standstill==1
    if update
        out=in;
    else
        out=inrecorder;
    end
end

== matlab function PvtSubSys_HMI/HMI2.12/IFC_Signal1/Subsystem25/MATLAB Function1 ==
  data: standstill input boolean; out output single; in input single; update input boolean; inrecorder input single; recorder output single
function [out,recorder] = fcn(standstill,in,update,inrecorder)
recorder=inrecorder;
out=single(0);
if update%当车辆由运动到静止时记录recorder，并在车辆运动时将recorder清零
    recorder=in;
end
if standstill==0%车辆运动时采用实际值，车辆静止时采用recorder值
    out=in;
elseif standstill==1
    if update
        out=in;
    else
        out=inrecorder;
    end
end

== matlab function PvtSubSys_HMI/HMI2.12/IFC_Signal1/Subsystem26/MATLAB Function1 ==
  data: standstill input boolean; out output single; in input single; update input boolean; inrecorder input single; recorder output single
function [out,recorder] = fcn(standstill,in,update,inrecorder)
recorder=inrecorder;
out=single(0);
if update%当车辆由运动到静止时记录recorder，并在车辆运动时将recorder清零
    recorder=in;
end
if standstill==0%车辆运动时采用实际值，车辆静止时采用recorder值
    out=in;
elseif standstill==1
    if update
        out=in;
    else
        out=inrecorder;
    end
end

== matlab function PvtSubSys_HMI/HMI2.12/IFC_Signal1/Subsystem27/MATLAB Function1 ==
  data: standstill input boolean; out output single; in input single; update input boolean; inrecorder input single; recorder output single
function [out,recorder] = fcn(standstill,in,update,inrecorder)
recorder=inrecorder;
out=single(0);
if update%当车辆由运动到静止时记录recorder，并在车辆运动时将recorder清零
    recorder=in;
end
if standstill==0%车辆运动时采用实际值，车辆静止时采用recorder值
    out=in;
elseif standstill==1
    if update
        out=in;
    else
        out=inrecorder;
    end
end

== matlab function PvtSubSys_HMI/HMI2.12/IFC_Signal1/Subsystem28/MATLAB Function1 ==
  data: standstill input boolean; out output single; in input single; update input boolean; inrecorder input single; recorder output single
function [out,recorder] = fcn(standstill,in,update,inrecorder)
recorder=inrecorder;
out=single(0);
if update%当车辆由运动到静止时记录recorder，并在车辆运动时将recorder清零
    recorder=in;
end
if standstill==0%车辆运动时采用实际值，车辆静止时采用recorder值
    out=in;
elseif standstill==1
    if update
        out=in;
    else
        out=inrecorder;
    end
end

== matlab function PvtSubSys_HMI/HMI2.12/IFC_Signal1/Subsystem29/MATLAB Function1 ==
  data: standstill input boolean; out output single; in input single; update input boolean; inrecorder input single; recorder output single
function [out,recorder] = fcn(standstill,in,update,inrecorder)
recorder=inrecorder;
out=single(0);
if update%当车辆由运动到静止时记录recorder，并在车辆运动时将recorder清零
    recorder=in;
end
if standstill==0%车辆运动时采用实际值，车辆静止时采用recorder值
    out=in;
elseif standstill==1
    if update
        out=in;
    else
        out=inrecorder;
    end
end

== matlab function PvtSubSys_HMI/HMI2.12/IFC_Signal1/Subsystem30/MATLAB Function1 ==
  data: standstill input boolean; out output single; in input single; update input boolean; inrecorder input single; recorder output single
function [out,recorder] = fcn(standstill,in,update,inrecorder)
recorder=inrecorder;
out=single(0);
if update%当车辆由运动到静止时记录recorder，并在车辆运动时将recorder清零
    recorder=in;
end
if standstill==0%车辆运动时采用实际值，车辆静止时采用recorder值
    out=in;
elseif standstill==1
    if update
        out=in;
    else
        out=inrecorder;
    end
end

== matlab function PvtSubSys_HMI/HMI2.12/HWA//ACC//TJA_Signal1/MATLAB Function ==
  data: ACCSts input; Longctrl_ModSts output; ACCStsK1 input; CntK1 input uint8; Cnt output
function [Longctrl_ModSts,Cnt]= fcn(ACCSts,ACCStsK1,CntK1)


if ((ACCStsK1==6||ACCStsK1==9)&&(ACCSts==7))
    Cnt = uint8(76);
else
    Cnt = max(CntK1 - uint8(1),uint8(1));
end

Longctrl_ModSts=ACCSts;
if ACCSts==6 || ACCSts==9
    Longctrl_ModSts=uint8(6);
elseif ACCSts==7 || Cnt>1
    if Cnt>6
        Longctrl_ModSts=uint8(7);
    else
        Longctrl_ModSts=uint8(0);
    end
end

== matlab function PvtSubSys_HMI/HMI2.12/IFC_Signal1/Subsystem31/MATLAB Function1 ==
  data: standstill input boolean; out output single; in input single; update input boolean; inrecorder input single; recorder output single
function [out,recorder] = fcn(standstill,in,update,inrecorder)
recorder=inrecorder;
out=single(0);
if update%当车辆由运动到静止时记录recorder，并在车辆运动时将recorder清零
    recorder=in;
end
if standstill==0%车辆运动时采用实际值，车辆静止时采用recorder值
    out=in;
elseif standstill==1
    if update
        out=in;
    else
        out=inrecorder;
    end
end

== matlab function PvtSubSys_HMI/HMI2.12/IFC_Signal1/Subsystem32/MATLAB Function1 ==
  data: standstill input boolean; out output single; in input single; update input boolean; inrecorder input single; recorder output single
function [out,recorder] = fcn(standstill,in,update,inrecorder)
recorder=inrecorder;
out=single(0);
if update%当车辆由运动到静止时记录recorder，并在车辆运动时将recorder清零
    recorder=in;
end
if standstill==0%车辆运动时采用实际值，车辆静止时采用recorder值
    out=in;
elseif standstill==1
    if update
        out=in;
    else
        out=inrecorder;
    end
end

== matlab function PvtSubSys_HMI/HMI2.12/IFC_Signal1/Subsystem33/MATLAB Function1 ==
  data: standstill input boolean; out output single; in input single; update input boolean; inrecorder input single; recorder output single
function [out,recorder] = fcn(standstill,in,update,inrecorder)
recorder=inrecorder;
out=single(0);
if update%当车辆由运动到静止时记录recorder，并在车辆运动时将recorder清零
    recorder=in;
end
if standstill==0%车辆运动时采用实际值，车辆静止时采用recorder值
    out=in;
elseif standstill==1
    if update
        out=in;
    else
        out=inrecorder;
    end
end

== matlab function PvtSubSys_HMI/HMI2.12/IFC_Signal1/Subsystem34/MATLAB Function1 ==
  data: standstill input boolean; out output single; in input single; update input boolean; inrecorder input single; recorder output single
function [out,recorder] = fcn(standstill,in,update,inrecorder)
recorder=inrecorder;
out=single(0);
if update%当车辆由运动到静止时记录recorder，并在车辆运动时将recorder清零
    recorder=in;
end
if standstill==0%车辆运动时采用实际值，车辆静止时采用recorder值
    out=in;
elseif standstill==1
    if update
        out=in;
    else
        out=inrecorder;
    end
end

== matlab function PvtSubSys_HMI/HMI2.12/IFC_Signal1/Subsystem35/MATLAB Function1 ==
  data: standstill input boolean; out output uint8; in input uint8; update input boolean; inrecorder input uint8; recorder output uint8
function [out,recorder] = fcn(standstill,in,update,inrecorder)
recorder=inrecorder;
out=uint8(0);
if update%当车辆由运动到静止时记录recorder，并在车辆运动时将recorder清零
    recorder=in;
end
if standstill==0%车辆运动时采用实际值，车辆静止时采用recorder值
    out=in;
elseif standstill==1
    if update
        out=in;
    else
        out=inrecorder;
    end
end

== matlab function PvtSubSys_HMI/HMI2.12/IFC_Signal1/Subsystem36/MATLAB Function1 ==
  data: standstill input boolean; out output single; in input single; update input boolean; inrecorder input single; recorder output single
function [out,recorder] = fcn(standstill,in,update,inrecorder)
recorder=inrecorder;
out=single(0);
if update%当车辆由运动到静止时记录recorder，并在车辆运动时将recorder清零
    recorder=in;
end
if standstill==0%车辆运动时采用实际值，车辆静止时采用recorder值
    out=in;
elseif standstill==1
    if update
        out=in;
    else
        out=inrecorder;
    end
end

== matlab function PvtSubSys_HMI/HMI2.12/IFC_Signal1/Subsystem37/MATLAB Function1 ==
  data: standstill input boolean; out output single; in input single; update input boolean; inrecorder input single; recorder output single
function [out,recorder] = fcn(standstill,in,update,inrecorder)
recorder=inrecorder;
out=single(0);
if update%当车辆由运动到静止时记录recorder，并在车辆运动时将recorder清零
    recorder=in;
end
if standstill==0%车辆运动时采用实际值，车辆静止时采用recorder值
    out=in;
elseif standstill==1
    if update
        out=in;
    else
        out=inrecorder;
    end
end

== matlab function PvtSubSys_HMI/HMI2.12/IFC_Signal1/Subsystem38/MATLAB Function1 ==
  data: standstill input boolean; out output single; in input single; update input boolean; inrecorder input single; recorder output single
function [out,recorder] = fcn(standstill,in,update,inrecorder)
recorder=inrecorder;
out=single(0);
if update%当车辆由运动到静止时记录recorder，并在车辆运动时将recorder清零
    recorder=in;
end
if standstill==0%车辆运动时采用实际值，车辆静止时采用recorder值
    out=in;
elseif standstill==1
    if update
        out=in;
    else
        out=inrecorder;
    end
end

== matlab function PvtSubSys_HMI/HMI2.12/IFC_Signal1/Subsystem39/MATLAB Function1 ==
  data: standstill input boolean; out output single; in input single; update input boolean; inrecorder input single; recorder output single
function [out,recorder] = fcn(standstill,in,update,inrecorder)
recorder=inrecorder;
out=single(0);
if update%当车辆由运动到静止时记录recorder，并在车辆运动时将recorder清零
    recorder=in;
end
if standstill==0%车辆运动时采用实际值，车辆静止时采用recorder值
    out=in;
elseif standstill==1
    if update
        out=in;
    else
        out=inrecorder;
    end
end

== matlab function PvtSubSys_HMI/HMI2.12/IFC_Signal1/Subsystem40/MATLAB Function1 ==
  data: standstill input boolean; out output uint8; in input uint8; update input boolean; inrecorder input uint8; recorder output uint8
function [out,recorder] = fcn(standstill,in,update,inrecorder)
recorder=inrecorder;
out=uint8(0);
if update%当车辆由运动到静止时记录recorder，并在车辆运动时将recorder清零
    recorder=in;
end
if standstill==0%车辆运动时采用实际值，车辆静止时采用recorder值
    out=in;
elseif standstill==1
    if update
        out=in;
    else
        out=inrecorder;
    end
end

== matlab function PvtSubSys_HMI/HMI2.12/HWA//ACC//TJA_Signal1/MATLAB Function1 ==
  data: ACCSts input; EgoStatus output; DecelReq input
function EgoStatus = fcn(ACCSts,DecelReq)
EgoStatus=uint8(0);
if ACCSts==5
    EgoStatus=uint8(1);
end
if DecelReq==1
    EgoStatus=uint8(2);
end

== matlab function PvtSubSys_HMI/HMI2.12/IFC_Signal1/Subsystem41/MATLAB Function1 ==
  data: standstill input boolean; out output single; in input single; update input boolean; inrecorder input single; recorder output single
function [out,recorder] = fcn(standstill,in,update,inrecorder)
recorder=inrecorder;
out=single(0);
if update%当车辆由运动到静止时记录recorder，并在车辆运动时将recorder清零
    recorder=in;
end
if standstill==0%车辆运动时采用实际值，车辆静止时采用recorder值
    out=in;
elseif standstill==1
    if update
        out=in;
    else
        out=inrecorder;
    end
end

== matlab function PvtSubSys_HMI/HMI2.12/IFC_Signal1/Subsystem42/MATLAB Function1 ==
  data: standstill input boolean; out output single; in input single; update input boolean; inrecorder input single; recorder output single
function [out,recorder] = fcn(standstill,in,update,inrecorder)
recorder=inrecorder;
out=single(0);
if update%当车辆由运动到静止时记录recorder，并在车辆运动时将recorder清零
    recorder=in;
end
if standstill==0%车辆运动时采用实际值，车辆静止时采用recorder值
    out=in;
elseif standstill==1
    if update
        out=in;
    else
        out=inrecorder;
    end
end

== matlab function PvtSubSys_HMI/HMI2.12/IFC_Signal1/Subsystem43/MATLAB Function1 ==
  data: standstill input boolean; out output single; in input single; update input boolean; inrecorder input single; recorder output single
function [out,recorder] = fcn(standstill,in,update,inrecorder)
recorder=inrecorder;
out=single(0);
if update%当车辆由运动到静止时记录recorder，并在车辆运动时将recorder清零
    recorder=in;
end
if standstill==0%车辆运动时采用实际值，车辆静止时采用recorder值
    out=in;
elseif standstill==1
    if update
        out=in;
    else
        out=inrecorder;
    end
end

== matlab function PvtSubSys_HMI/HMI2.12/IFC_Signal1/Subsystem44/MATLAB Function1 ==
  data: standstill input boolean; out output single; in input single; update input boolean; inrecorder input single; recorder output single
function [out,recorder] = fcn(standstill,in,update,inrecorder)
recorder=inrecorder;
out=single(0);
if update%当车辆由运动到静止时记录recorder，并在车辆运动时将recorder清零
    recorder=in;
end
if standstill==0%车辆运动时采用实际值，车辆静止时采用recorder值
    out=in;
elseif standstill==1
    if update
        out=in;
    else
        out=inrecorder;
    end
end

== matlab function PvtSubSys_HMI/HMI2.12/IFC_Signal1/Subsystem45/MATLAB Function1 ==
  data: standstill input boolean; out output single; in input single; update input boolean; inrecorder input single; recorder output single
function [out,recorder] = fcn(standstill,in,update,inrecorder)
recorder=inrecorder;
out=single(0);
if update%当车辆由运动到静止时记录recorder，并在车辆运动时将recorder清零
    recorder=in;
end
if standstill==0%车辆运动时采用实际值，车辆静止时采用recorder值
    out=in;
elseif standstill==1
    if update
        out=in;
    else
        out=inrecorder;
    end
end

== matlab function PvtSubSys_HMI/HMI2.12/IFC_Signal1/Subsystem46/MATLAB Function1 ==
  data: standstill input boolean; out output single; in input single; update input boolean; inrecorder input single; recorder output single
function [out,recorder] = fcn(standstill,in,update,inrecorder)
recorder=inrecorder;
out=single(0);
if update%当车辆由运动到静止时记录recorder，并在车辆运动时将recorder清零
    recorder=in;
end
if standstill==0%车辆运动时采用实际值，车辆静止时采用recorder值
    out=in;
elseif standstill==1
    if update
        out=in;
    else
        out=inrecorder;
    end
end

== matlab function PvtSubSys_HMI/HMI2.12/IFC_Signal1/Subsystem47/MATLAB Function1 ==
  data: standstill input boolean; out output single; in input single; update input boolean; inrecorder input single; recorder output single
function [out,recorder] = fcn(standstill,in,update,inrecorder)
recorder=inrecorder;
out=single(0);
if update%当车辆由运动到静止时记录recorder，并在车辆运动时将recorder清零
    recorder=in;
end
if standstill==0%车辆运动时采用实际值，车辆静止时采用recorder值
    out=in;
elseif standstill==1
    if update
        out=in;
    else
        out=inrecorder;
    end
end

== matlab function PvtSubSys_HMI/HMI2.12/HWA//ACC//TJA_Signal1/MATLAB Function2 ==
  data: TJA_ACC_SelSts input; y output
function y = fcn(TJA_ACC_SelSts)
y=TJA_ACC_SelSts;
if TJA_ACC_SelSts==3
    y=uint8(0);
elseif TJA_ACC_SelSts==0
    y=uint8(3);
end

== matlab function PvtSubSys_HMI/HMI2.12/IFC_Signal1/Subsystem48/MATLAB Function1 ==
  data: standstill input boolean; out output single; in input single; update input boolean; inrecorder input single; recorder output single
function [out,recorder] = fcn(standstill,in,update,inrecorder)
recorder=inrecorder;
out=single(0);
if update%当车辆由运动到静止时记录recorder，并在车辆运动时将recorder清零
    recorder=in;
end
if standstill==0%车辆运动时采用实际值，车辆静止时采用recorder值
    out=in;
elseif standstill==1
    if update
        out=in;
    else
        out=inrecorder;
    end
end

== matlab function PvtSubSys_HMI/HMI2.12/IFC_Signal1/Subsystem49/MATLAB Function1 ==
  data: standstill input boolean; out output single; in input single; update input boolean; inrecorder input single; recorder output single
function [out,recorder] = fcn(standstill,in,update,inrecorder)
recorder=inrecorder;
out=single(0);
if update%当车辆由运动到静止时记录recorder，并在车辆运动时将recorder清零
    recorder=in;
end
if standstill==0%车辆运动时采用实际值，车辆静止时采用recorder值
    out=in;
elseif standstill==1
    if update
        out=in;
    else
        out=inrecorder;
    end
end
